simulink model "milestonetwo_oldsetup"  (R2025a)
settings: Solver=FixedStepAuto  StartTime=0.0  StopTime=10  FixedStep=1e-3  RelTol=1e-3  EnableMultiTasking=on
model workspace (MAT data in the model file):
  Var = 0
  x = 1
undefined symbols (not defined in the file): D0, D1, D10, D11, D12, D13, D2, D3, D5, D6, D8, D9, PTA0, PTA1, PTA2, PTB9, PTC16, PTC17, PTC2, PTC4, PTD0, PTD1, PTD2, PTD3
libraries: frdmk64flib x14
settings Model: ExtModeTrigDuration=5  Creator=alber  LastModifiedBy=ybakr
settings OptimizationCC: BlockReduction=off  DefaultParameterBehavior=Inlined  BufferReuse=off  EnhancedBackFolding=on  PassReuseOutputArgsAs=Individual arguments  ZeroExternalMemoryAtStartup=off  ZeroInternalMemoryAtStartup=off  MaxStackSize=64  OptimizeBlockOrder=speed  DifferentSizesBufferReuse=on  EfficientTunableParamExpr=on
settings DebuggingCC: ParameterTunabilityLossMsg=error
settings HardwareCC: ProdBitPerPointer=32.0  ProdBitPerSizeT=32.0  ProdBitPerPtrDiffT=32.0  ProdLargestAtomicInteger=Long  ProdLargestAtomicFloat=Double  ProdWordSize=32.0  ProdHWDeviceType=ARM Compatible->ARM Cortex
settings SFSimCC: MATLABDynamicMemAlloc=off
settings RTWCC: SystemTargetFile=ert.tlc  HardwareBoard=NXP FRDM-K64F  TLCOptions="-aInlineSetEventsForThisBaseRateFcn=TLC_FALSE -aSuppressMultiTaskScheduler=TLC_FALSE  -aRateBasedStepFcn=0"  TemplateMakefile=ert_default_tmf  Toolchain=GNU Tools for ARM Embedded Processors  Description=Embedded Coder
settings CodeAppCC: ForceParamTrailComments=on  IgnoreCustomStorageClasses=off  OperatorAnnotations=on  SimulinkDataObjDesc=on  SFDataObjDesc=on  InsertBlockDesc=on
settings ERTTargetCC: ExtModeTransport=4.0  ExtModeStaticAlloc=off  ExtModeMexFile=sendToCommService  ExtModeIntrfLevel=Level1

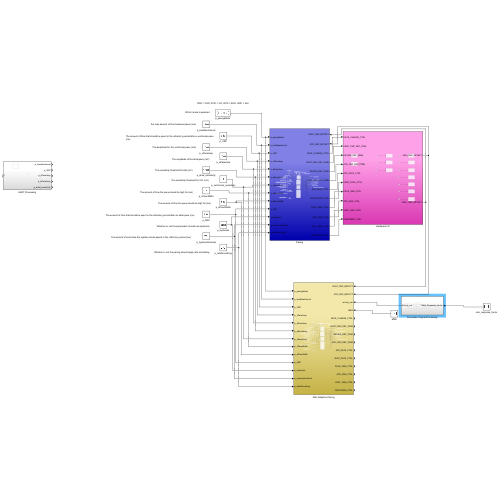
[thumbnail: Simulink's stored preview of the top-level diagram]
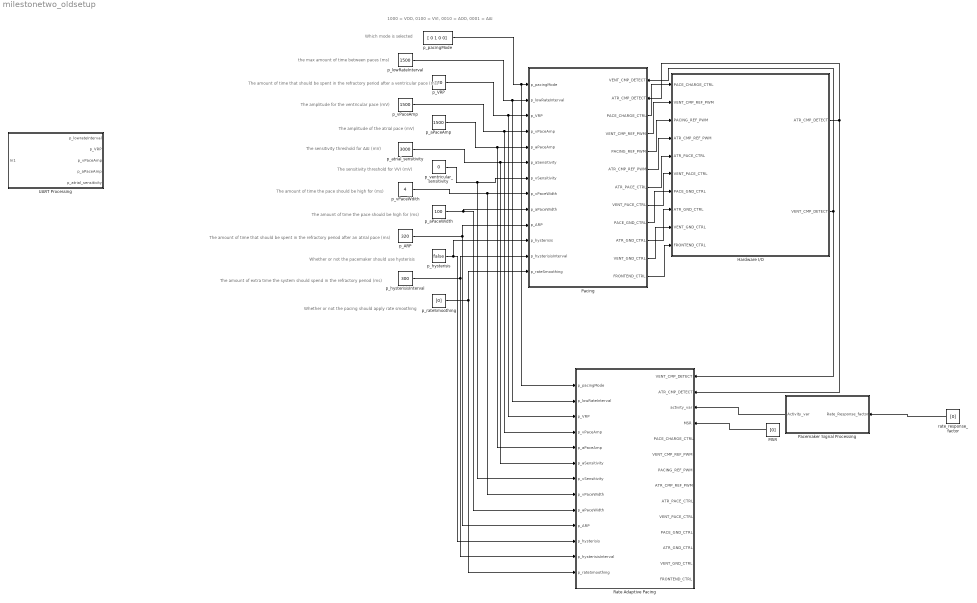
== system milestonetwo_oldsetup ==
  note: The amount of extra time the system should spend in the refractory period (ms)
  note: Whether or not the pacemaker should use hysterisis
  note: Whether or not the pacing should apply rate smoothing
  note: The amplitude of the atrial pace (mV)
  note: The sensitivity threshold for VVI (mV)
  note: The amount of time that should be spent in the refractory period after a ventricular pace (ms)
  note: The amount of time the pace should be high for (ms)
  note: The amplitude for the ventricular pace (mV)
  note: the max amount of time between paces (ms)
  note: Which mode is selected
  note: 1000 = VOO, 0100 = VVI, 0010 = AOO, 0001 = AAI
  note: The amount of time the pace should be high for (ms)
  note: The sensitivity threshold for AAI (mV)
  note: The amount of time that should be spent in the refractory period after an atrial pace (ms)
  Hardware I/O : Subsystem
  MSR : Constant  Value=[0]  OutDataTypeStr=uint16
  Pacemaker Signal Processing : Subsystem
  Pacing : Subsystem
      settings: PortSchema="{\"entries\":[{\"content\":{\"sides\":[{\"content\":{\"connectorIds\":[\"In1\",\"In2\",\"In3\",\"In4\",\"In5\",\"In6\",\"In7\",\"In8\",\"In9\",\"In10\",\"In11\",\"In12\",\"In13\"]},\"type\":\"ConnectorPlacement.EquallySpacedRectSide\",\"uuid\":\"83755f54-be08-4212-abd8-522318738612\"},{\"content\":{\"connectorIds\":[\"In14\",\"In15\",\"Out1\",\"Out2\",\"Out3\",\"Out4\",\"Out5\",\"Out6\",\"Out7\",\"Out8\",\"Out9\",\"Out10\"],\"side\":\"RIGHT\"},\"type\":\"ConnectorPlacement.EquallySpacedRectSide\",\"uuid\":\"fddfc3a4-50da-418e-a4c1-261999e6a94a\"},{\"content\":{\"side\":\"TOP\"},\"type\":\"ConnectorPlacement.EquallySpacedRectSide\",\"uuid\":\"96bf6691-7ea4-44be-8ce9-22c29429ec55\"}]},\"type\":\"ConnectorPlacement.EquallySpacedConnector\",\"uuid\":\"94865ebc-bf15-4e1f-8273-6a484a8d613b\"}],\"packageUris\":[\"http://schema.mathworks.com/mf0/Connector/R2020b\"],\"version\":\"1.0\"}"
  Rate Adaptive Pacing : Subsystem
      settings: PortSchema="{\"entries\":[{\"content\":{\"sides\":[{\"content\":{\"connectorIds\":[\"In1\",\"In2\",\"In3\",\"In4\",\"In5\",\"In6\",\"In7\",\"In8\",\"In9\",\"In10\",\"In11\",\"In12\",\"In13\"]},\"type\":\"ConnectorPlacement.EquallySpacedRectSide\",\"uuid\":\"83755f54-be08-4212-abd8-522318738612\"},{\"content\":{\"connectorIds\":[\"In14\",\"In15\",\"In16\",\"In17\",\"Out1\",\"Out2\",\"Out3\",\"Out4\",\"Out5\",\"Out6\",\"Out7\",\"Out8\",\"Out9\",\"Out10\"],\"side\":\"RIGHT\"},\"type\":\"ConnectorPlacement.EquallySpacedRectSide\",\"uuid\":\"fddfc3a4-50da-418e-a4c1-261999e6a94a\"},{\"content\":{\"side\":\"TOP\"},\"type\":\"ConnectorPlacement.EquallySpacedRectSide\",\"uuid\":\"96bf6691-7ea4-44be-8ce9-22c29429ec55\"}]},\"type\":\"ConnectorPlacement.EquallySpacedConnector\",\"uuid\":\"94865ebc-bf15-4e1f-8273-6a484a8d613b\"}],\"packageUris\":[\"http://schema.mathworks.com/mf0/Connector/R2020b\"],\"version\":\"1.0\"}"
  UART Processing : Subsystem
  p_ARP : Constant  Value=320  OutMin=[150]  OutMax=[500]  OutDataTypeStr=uint16
  p_VRP : Constant  Value=320  OutMin=[150]  OutMax=[500]  OutDataTypeStr=uint16
  p_aPaceAmp : Constant  Value=1500  OutDataTypeStr=uint16
  p_aPaceWidth : Constant  Value=100  OutDataTypeStr=int16
  p_atrial_sensitivity : Constant  Value=3000  OutDataTypeStr=uint16
  p_hysterisis : Constant  Value=false  OutDataTypeStr=uint16
  p_hysterisisInterval : Constant  Value=300  OutDataTypeStr=uint16
  p_lowRateInterval : Constant  Value=1500  OutMin=[343]  OutMax=[2000]  OutDataTypeStr=uint16
  p_pacingMode : Constant  Value=[ 0 1 0 0]  OutDataTypeStr=uint8
  p_rateSmoothing : Constant  Value=[0]  OutDataTypeStr=uint16
  p_vPaceAmp : Constant  Value=1500  OutMin=[500]  OutMax=[7000]  OutDataTypeStr=uint16
  p_vPaceWdith : Constant  Value=4  OutMin=[1]  OutMax=[19]  OutDataTypeStr=int16
  p_ventricular_sensitivity : Constant  Value=0  OutDataTypeStr=uint16
  rate_response_factor : Constant  Value=[0]  OutDataTypeStr=uint16
  wires:
  p_pacingMode/1 -> Rate Adaptive Pacing/1(p_pacingMode), Pacing/1(p_pacingMode)
  p_aPaceWidth/1 -> Rate Adaptive Pacing/9(p_aPaceWidth), Pacing/9(p_aPaceWidth)
  p_aPaceAmp/1 -> Rate Adaptive Pacing/5(p_aPaceAmp), Pacing/5(p_aPaceAmp)
  p_lowRateInterval/1 -> Rate Adaptive Pacing/2(p_lowRateInterval), Pacing/2(p_lowRateInterval)
  p_vPaceAmp/1 -> Rate Adaptive Pacing/4(p_vPaceAmp), Pacing/4(p_vPaceAmp)
  p_vPaceWdith/1 -> Rate Adaptive Pacing/8(p_vPaceWidth), Pacing/8(p_vPaceWidth)
  p_hysterisis/1 -> Rate Adaptive Pacing/11(p_hysterisis), Pacing/11(p_hysterisis)
  p_hysterisisInterval/1 -> Rate Adaptive Pacing/12(p_hysterisisInterval), Pacing/12(p_hysterisisInterval)
  p_rateSmoothing/1 -> Pacing/13(p_rateSmoothing), Rate Adaptive Pacing/13(p_rateSmoothing)
  Pacing/1(PACE_CHARGE_CTRL) -> Hardware I/O/1(PACE_CHARGE_CTRL)
  p_VRP/1 -> Rate Adaptive Pacing/3(p_VRP), Pacing/3(p_VRP)
  p_ARP/1 -> Rate Adaptive Pacing/10(p_ARP), Pacing/10(p_ARP)
  Pacing/2(VENT_CMP_REF_PWM) -> Hardware I/O/2(VENT_CMP_REF_PWM)
  Pacing/3(PACING_REF_PWM) -> Hardware I/O/3(PACING_REF_PWM)
  Pacing/4(ATR_CMP_REF_PWM) -> Hardware I/O/4(ATR_CMP_REF_PWM)
  Pacing/10(FRONTEND_CTRL) -> Hardware I/O/10(FRONTEND_CTRL)
  Pacing/9(VENT_GND_CTRL) -> Hardware I/O/9(VENT_GND_CTRL)
  Pacing/8(ATR_GND_CTRL) -> Hardware I/O/8(ATR_GND_CTRL)
  Pacing/7(PACE_GND_CTRL) -> Hardware I/O/7(PACE_GND_CTRL)
  Pacing/6(VENT_PACE_CTRL) -> Hardware I/O/6(VENT_PACE_CTRL)
  Pacing/5(ATR_PACE_CTRL) -> Hardware I/O/5(ATR_PACE_CTRL)
  Hardware I/O/1(ATR_CMP_DETECT) -> Pacing/15(ATR_CMP_DETECT), Rate Adaptive Pacing/15(ATR_CMP_DETECT)
  Hardware I/O/2(VENT_CMP_DETECT) -> Pacing/14(VENT_CMP_DETECT), Rate Adaptive Pacing/14(VENT_CMP_DETECT)
  p_atrial_sensitivity/1 -> Rate Adaptive Pacing/6(p_aSensitivity), Pacing/6(p_aSensitivity)
  p_ventricular_sensitivity/1 -> Rate Adaptive Pacing/7(p_vSensitivity), Pacing/7(p_vSensitivity)
  rate_response_factor/1 -> Pacemaker Signal Processing/1(Rate_Response_factor)
  Pacemaker Signal Processing/1(Activity_var) -> Rate Adaptive Pacing/16(activity_var)
  MSR/1 -> Rate Adaptive Pacing/17(MSR)

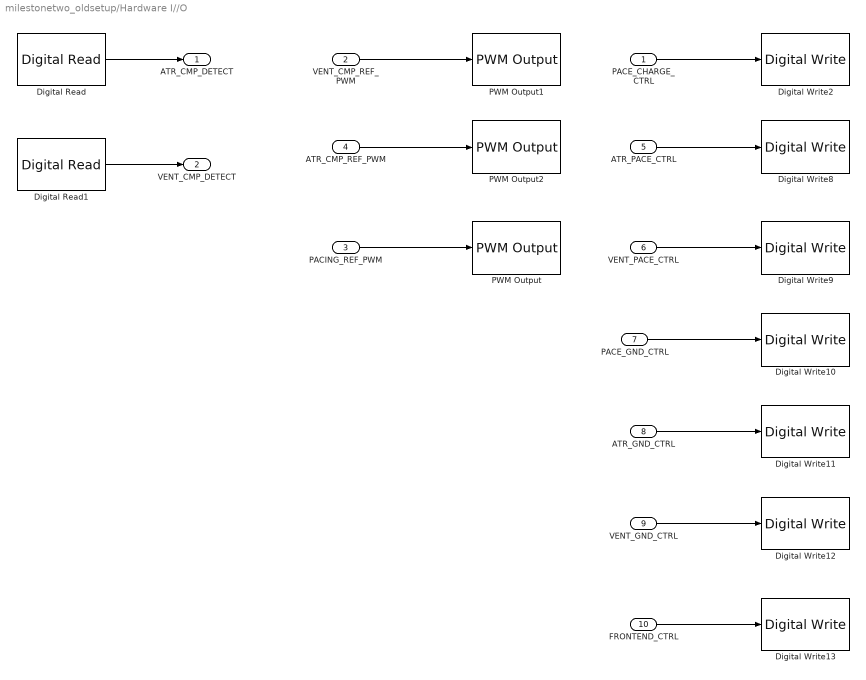
== system milestonetwo_oldsetup/Hardware I//O ==
  PACE_CHARGE_CTRL : Inport
  VENT_CMP_REF_PWM : Inport  Port=2
  PACING_REF_PWM : Inport  Port=3
  ATR_CMP_REF_PWM : Inport  Port=4
  ATR_PACE_CTRL : Inport  Port=5
  VENT_PACE_CTRL : Inport  Port=6
  PACE_GND_CTRL : Inport  Port=7
  ATR_GND_CTRL : Inport  Port=8
  VENT_GND_CTRL : Inport  Port=9
  FRONTEND_CTRL : Inport  Port=10
  Digital Read : frdmk64flib/Digital Read  Whichpin=PTC16 (D0)  SampleTime=-1
  Digital Read1 : frdmk64flib/Digital Read  Whichpin=PTC17 (D1)  SampleTime=-1
  Digital Write10 : frdmk64flib/Digital Write  Whichpin=PTD0 (D10)
  Digital Write11 : frdmk64flib/Digital Write  Whichpin=PTD2 (D11)
  Digital Write12 : frdmk64flib/Digital Write  Whichpin=PTD3 (D12)
  Digital Write13 : frdmk64flib/Digital Write  Whichpin=PTD1 (D13)
  Digital Write2 : frdmk64flib/Digital Write  Whichpin=PTB9 (D2)
  Digital Write8 : frdmk64flib/Digital Write  Whichpin=PTA0 (D8)
  Digital Write9 : frdmk64flib/Digital Write  Whichpin=PTC4 (D9)
  PWM Output : frdmk64flib/PWM Output  Whichpin=PTA2 (D5)  InitialFrequency=2000  InitialDutyCycle=0
  PWM Output1 : frdmk64flib/PWM Output  Whichpin=PTA1 (D3)  InitialFrequency=2000  InitialDutyCycle=0
  PWM Output2 : frdmk64flib/PWM Output  Whichpin=PTC2 (D6)  InitialFrequency=2000  InitialDutyCycle=0
  ATR_CMP_DETECT : Outport
  VENT_CMP_DETECT : Outport  Port=2
  wires:
  PACE_CHARGE_CTRL/1 -> Digital Write2/1
  PACING_REF_PWM/1 -> PWM Output/1
  VENT_CMP_REF_PWM/1 -> PWM Output1/1
  ATR_GND_CTRL/1 -> Digital Write11/1
  ATR_PACE_CTRL/1 -> Digital Write8/1
  VENT_PACE_CTRL/1 -> Digital Write9/1
  ATR_CMP_REF_PWM/1 -> PWM Output2/1
  VENT_GND_CTRL/1 -> Digital Write12/1
  FRONTEND_CTRL/1 -> Digital Write13/1
  Digital Read/1 -> ATR_CMP_DETECT/1
  Digital Read1/1 -> VENT_CMP_DETECT/1
  PACE_GND_CTRL/1 -> Digital Write10/1

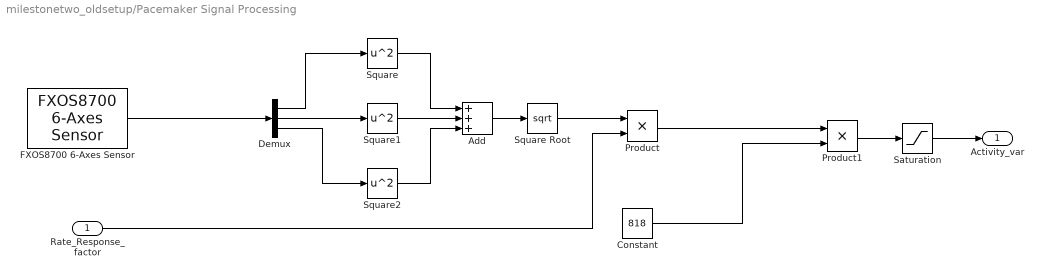
== system milestonetwo_oldsetup/Pacemaker Signal Processing ==
  Rate_Response_factor : Inport
  Add : Sum  Inputs=+++
  Constant : Constant  Value=818
  Demux : Demux  Outputs=3
  FXOS8700 6-Axes Sensor : frdmk64flib/FXOS8700 6-Axes Sensor  Activesensor=Accelerometer only  ODR=400Hz  HybridODR=400Hz  Accelfullrange=-4g to +4g  SampleTime=-1
  Product : Product
  Product1 : Product
  Saturation : Saturate  UpperLimit=7200  LowerLimit=1500
  Square : Math  Operator=square
  Square Root : Sqrt
  Square1 : Math  Operator=square
  Square2 : Math  Operator=square
  Activity_var : Outport
  wires:
  FXOS8700 6-Axes Sensor/1 -> Demux/1
  Rate_Response_factor/1 -> Product/2
  Demux/1 -> Square/1
  Demux/2 -> Square1/1
  Demux/3 -> Square2/1
  Square/1 -> Add/1
  Square1/1 -> Add/2
  Square2/1 -> Add/3
  Add/1 -> Square Root/1
  Square Root/1 -> Product/1
  Product/1 -> Product1/1
  Constant/1 -> Product1/2
  Product1/1 -> Saturation/1
  Saturation/1 -> Activity_var/1

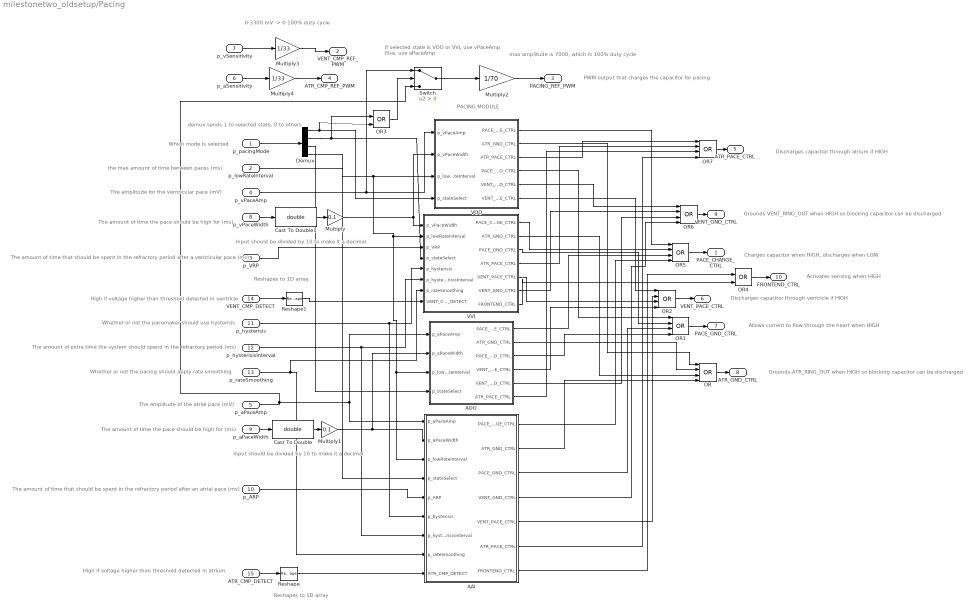
== system milestonetwo_oldsetup/Pacing ==
  note: Activates sensing when HIGH
  note: Charges capacitor when HIGH, discharges when LOW
  note: Allows current to flow through the heart when HIGH
  note: Grounds ATR_RING_OUT when HIGH so blocking capacitor can be discharged
  note: Discharges capacitor through ventricle if HIGH
  note: Grounds VENT_RING_OUT when HIGH so blocking capacitor can be discharged
  note: Discharges capacitor through atrium if HIGH
  note: PWM output that charges the capacitor for pacing
  note: High if voltage higher than threshold detected in atrium
  note: Input should be divided by 10 to make it a decimal
  note: Reshapes to 1D array
  note: demux sends 1 to selected state, 0 to others
  note: If selected state is VOO or VVI, use vPaceAmp
      | Else, use aPaceAmp
  note: max amplitude is 7000, which is 100% duty cycle
  note: 0-3300 mV -> 0-100% duty cycle
  note: PACING MODULE
  note: Reshapes to 1D array
  note: Input should be divided by 10 to make it a decimal
  note: Whether or not the pacing should apply rate smoothing
  note: the max amount of time between paces (ms)
  note: The amount of extra time the system should spend in the refractory period (ms)
  note: High if voltage higher than threshold detected in ventricle
  note: The amount of time the pace should be high for (ms)
  note: The amount of time the pace should be high for (ms)
  note: The amplitude of the atrial pace (mV)
  note: The amount of time that should be spent in the refractory period after a ventricular pace (ms)
  note: Whether or not the pacemaker should use hysterisis
  note: The amplitude for the ventricular pace (mV)
  note: The amount of time that should be spent in the refractory period after an atrial pace (ms)
  note: Which mode is selected
  p_pacingMode : Inport
  p_lowRateInterval : Inport  Port=2
  p_VRP : Inport  Port=3
  p_vPaceAmp : Inport  Port=4
  p_aPaceAmp : Inport  Port=5
  p_aSensitivity : Inport  Port=6
  p_vSensitivity : Inport  Port=7
  p_vPaceWidth : Inport  Port=8
  p_aPaceWidth : Inport  Port=9
  p_ARP : Inport  Port=10
  p_hysterisis : Inport  Port=11
  p_hysterisisInterval : Inport  Port=12
  p_rateSmoothing : Inport  Port=13
  VENT_CMP_DETECT : Inport  Port=14  OutDataTypeStr=boolean
  ATR_CMP_DETECT : Inport  Port=15  OutDataTypeStr=boolean
  AAI : Stateflow chart  TreatAsAtomicUnit=on
      settings: PortSchema="{\"entries\":[{\"content\":{\"sides\":[{\"content\":{\"connectorIds\":[\"In5\",\"In1\",\"In2\",\"In3\",\"In4\",\"In6\",\"In7\",\"In8\",\"In9\"]},\"type\":\"ConnectorPlacement.EquallySpacedRectSide\",\"uuid\":\"cccc9f32-b255-4089-8202-5f4b6cf4849a\"},{\"content\":{\"connectorIds\":[\"Out1\",\"Out2\",\"Out3\",\"Out4\",\"Out5\",\"Out6\",\"Out7\"],\"side\":\"RIGHT\"},\"type\":\"ConnectorPlacement.EquallySpacedRectSide\",\"uuid\":\"983a4a60-3d5c-4e53-84aa-b68c0bc6099e\"},{\"content\":{\"side\":\"TOP\"},\"type\":\"ConnectorPlacement.EquallySpacedRectSide\",\"uuid\":\"2756b790-cbb9-4039-b4f9-91cb14419ddd\"}]},\"type\":\"ConnectorPlacement.EquallySpacedConnector\",\"uuid\":\"1ccddf37-9dbc-46c0-8904-a3b9c6a38aa8\"}],\"packageUris\":[\"http://schema.mathworks.com/mf0/Connector/R2020b\"],\"version\":\"1.0\"}"
  AOO : Stateflow chart  TreatAsAtomicUnit=on
  Cast To Double : DataTypeConversion  OutDataTypeStr=double  SaturateOnIntegerOverflow=off  RndMeth=Floor
  Cast To Double1 : DataTypeConversion  OutDataTypeStr=double  SaturateOnIntegerOverflow=off  RndMeth=Floor
  Demux : Demux
  Multiply : Gain  Gain=0.1
  Multiply1 : Gain  Gain=0.1
  Multiply2 : Gain  Gain=1/70
  Multiply3 : Gain  Gain=1/33
  Multiply4 : Gain  Gain=1/33
  OR{,1..2,5..7} (6 alike) : Logic  Operator=OR  Inputs=4  IconShape=distinctive  AllPortsSameDT=off  OutDataTypeStr=boolean
  OR3 : Logic  Operator=OR  IconShape=distinctive  AllPortsSameDT=off  OutDataTypeStr=boolean
  OR4 : Logic  Operator=OR  IconShape=distinctive  AllPortsSameDT=off  OutDataTypeStr=boolean
  Reshape : Reshape
  Reshape1 : Reshape
  Switch : Switch  Criteria=u2 > Threshold  SaturateOnIntegerOverflow=off  InputSameDT=off
  VOO : Stateflow chart  TreatAsAtomicUnit=on
  VVI : Stateflow chart  TreatAsAtomicUnit=on
  PACE_CHARGE_CTRL : Outport
  VENT_CMP_REF_PWM : Outport  Port=2
  PACING_REF_PWM : Outport  Port=3
  ATR_CMP_REF_PWM : Outport  Port=4
  ATR_PACE_CTRL : Outport  Port=5
  VENT_PACE_CTRL : Outport  Port=6
  PACE_GND_CTRL : Outport  Port=7
  ATR_GND_CTRL : Outport  Port=8
  VENT_GND_CTRL : Outport  Port=9
  FRONTEND_CTRL : Outport  Port=10
  wires:
  Multiply/1 -> VVI/1(p_vPaceWidth), VOO/2(p_vPaceWidth)
  Multiply1/1 -> AAI/1(p_aPaceWidth), AOO/2(p_aPaceWidth)
  Cast To Double1/1 -> Multiply/1
  Cast To Double/1 -> Multiply1/1
  p_aPaceWidth/1 -> Cast To Double/1
  p_vPaceWidth/1 -> Cast To Double1/1
  p_lowRateInterval/1 -> AAI/2(p_lowRateInterval), AOO/3(p_lowRateInterval), VVI/2(p_lowRateInterval), VOO/3(p_lowRateInterval)
  p_ARP/1 -> AAI/4(p_ARP)
  p_VRP/1 -> VVI/3(p_VRP)
  p_hysterisis/1 -> AAI/6(p_hysterisis), VVI/5(p_hysterisis)
  p_hysterisisInterval/1 -> VVI/6(p_hysterisisInterval), AAI/7(p_hysterisisInterval)
  p_rateSmoothing/1 -> VVI/7(p_rateSmoothing), AAI/8(p_rateSmoothing)
  p_pacingMode/1 -> Demux/1
  Demux/1 -> OR3/2, VOO/4(p_stateSelect)
  Demux/2 -> OR3/1, VVI/4(p_stateSelect)
  Demux/3 -> AOO/4(p_stateSelect)
  Demux/4 -> AAI/3(p_stateSelect)
  p_vPaceAmp/1 -> Switch/1, VOO/1(p_vPaceAmp)
  p_aPaceAmp/1 -> AOO/1(p_aPaceAmp), AAI/5(p_aPaceAmp), Switch/3
  VOO/1(PACE_CHARGE_CTRL) -> OR5/1
  VVI/1(PACE_CHARGE_CTRL) -> OR5/2
  AOO/1(PACE_CHARGE_CTRL) -> OR5/3
  AAI/1(PACE_CHARGE_CTRL) -> OR5/4
  VOO/3(ATR_PACE_CTRL) -> OR7/1
  VVI/4(ATR_PACE_CTRL) -> OR7/2
  AOO/6(ATR_PACE_CTRL) -> OR7/3
  AOO/4(VENT_PACE_CTRL) -> OR2/4
  AAI/5(VENT_PACE_CTRL) -> OR2/2
  VVI/5(VENT_PACE_CTRL) -> OR2/3
  VOO/6(VENT_PACE_CTRL) -> OR2/1
  AAI/3(PACE_GND_CTRL) -> OR1/3
  AOO/3(PACE_GND_CTRL) -> OR1/4
  VVI/3(PACE_GND_CTRL) -> OR1/2
  VOO/4(PACE_GND_CTRL) -> OR1/1
  AAI/2(ATR_GND_CTRL) -> OR/4
  AOO/2(ATR_GND_CTRL) -> OR/2
  VVI/2(ATR_GND_CTRL) -> OR/3
  VOO/2(ATR_GND_CTRL) -> OR/1
  VOO/5(VENT_GND_CTRL) -> OR6/1
  VVI/6(VENT_GND_CTRL) -> OR6/2
  AOO/5(VENT_GND_CTRL) -> OR6/3
  AAI/4(VENT_GND_CTRL) -> OR6/4
  VVI/7(FRONTEND_CTRL) -> OR4/2
  AAI/7(FRONTEND_CTRL) -> OR4/1
  ATR_CMP_DETECT/1 -> Reshape/1
  VENT_CMP_DETECT/1 -> Reshape1/1
  Multiply2/1 -> PACING_REF_PWM/1
  Reshape/1 -> AAI/9(ATR_CMP_DETECT)
  Reshape1/1 -> VVI/8(VENT_CMP_DETECT)
  OR/1 -> ATR_GND_CTRL/1
  OR1/1 -> PACE_GND_CTRL/1
  OR2/1 -> VENT_PACE_CTRL/1
  OR3/1 -> Switch/2
  OR4/1 -> FRONTEND_CTRL/1
  OR5/1 -> PACE_CHARGE_CTRL/1
  OR6/1 -> VENT_GND_CTRL/1
  AAI/6(ATR_PACE_CTRL) -> OR7/4
  OR7/1 -> ATR_PACE_CTRL/1
  p_vSensitivity/1 -> Multiply3/1
  Multiply3/1 -> VENT_CMP_REF_PWM/1
  p_aSensitivity/1 -> Multiply4/1
  Multiply4/1 -> ATR_CMP_REF_PWM/1
  Switch/1 -> Multiply2/1

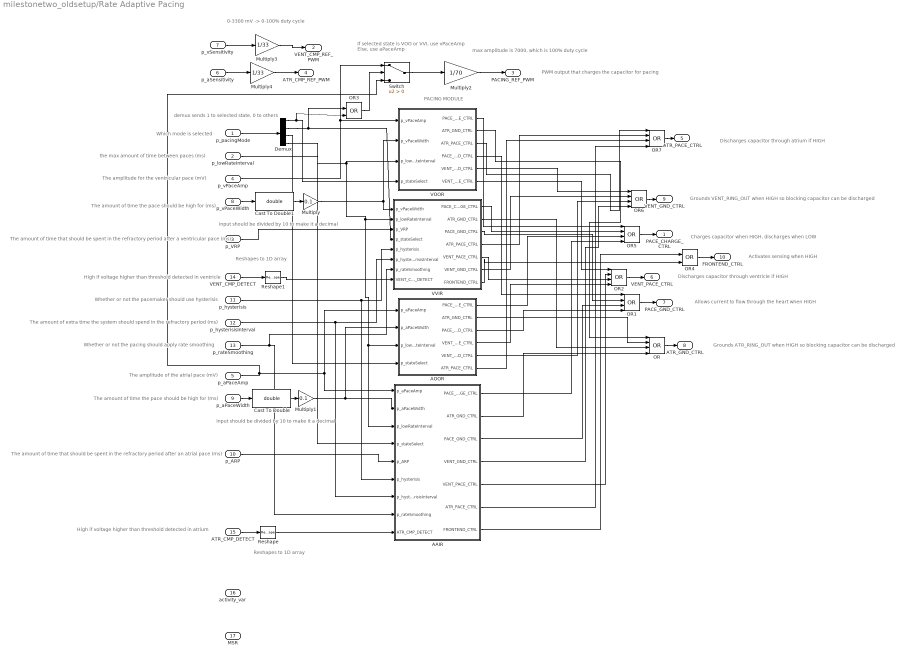
== system milestonetwo_oldsetup/Rate Adaptive Pacing ==
  note: Activates sensing when HIGH
  note: Charges capacitor when HIGH, discharges when LOW
  note: Allows current to flow through the heart when HIGH
  note: Grounds ATR_RING_OUT when HIGH so blocking capacitor can be discharged
  note: Discharges capacitor through ventricle if HIGH
  note: Grounds VENT_RING_OUT when HIGH so blocking capacitor can be discharged
  note: Discharges capacitor through atrium if HIGH
  note: PWM output that charges the capacitor for pacing
  note: High if voltage higher than threshold detected in atrium
  note: Input should be divided by 10 to make it a decimal
  note: Reshapes to 1D array
  note: demux sends 1 to selected state, 0 to others
  note: If selected state is VOO or VVI, use vPaceAmp
      | Else, use aPaceAmp
  note: max amplitude is 7000, which is 100% duty cycle
  note: 0-3300 mV -> 0-100% duty cycle
  note: PACING MODULE
  note: Reshapes to 1D array
  note: Input should be divided by 10 to make it a decimal
  note: Whether or not the pacing should apply rate smoothing
  note: the max amount of time between paces (ms)
  note: The amount of extra time the system should spend in the refractory period (ms)
  note: High if voltage higher than threshold detected in ventricle
  note: The amount of time the pace should be high for (ms)
  note: The amount of time the pace should be high for (ms)
  note: The amplitude of the atrial pace (mV)
  note: The amount of time that should be spent in the refractory period after a ventricular pace (ms)
  note: Whether or not the pacemaker should use hysterisis
  note: The amplitude for the ventricular pace (mV)
  note: The amount of time that should be spent in the refractory period after an atrial pace (ms)
  note: Which mode is selected
  p_pacingMode : Inport
  p_lowRateInterval : Inport  Port=2
  p_VRP : Inport  Port=3
  p_vPaceAmp : Inport  Port=4
  p_aPaceAmp : Inport  Port=5
  p_aSensitivity : Inport  Port=6
  p_vSensitivity : Inport  Port=7
  p_vPaceWidth : Inport  Port=8
  p_aPaceWidth : Inport  Port=9
  p_ARP : Inport  Port=10
  p_hysterisis : Inport  Port=11
  p_hysterisisInterval : Inport  Port=12
  p_rateSmoothing : Inport  Port=13
  VENT_CMP_DETECT : Inport  Port=14  OutDataTypeStr=boolean
  ATR_CMP_DETECT : Inport  Port=15  OutDataTypeStr=boolean
  activity_var : Inport  Port=16  OutDataTypeStr=boolean
  MSR : Inport  Port=17  OutDataTypeStr=boolean
  AAIR : Stateflow chart  TreatAsAtomicUnit=on
      settings: PortSchema="{\"entries\":[{\"content\":{\"sides\":[{\"content\":{\"connectorIds\":[\"In5\",\"In1\",\"In2\",\"In3\",\"In4\",\"In6\",\"In7\",\"In8\",\"In9\"]},\"type\":\"ConnectorPlacement.EquallySpacedRectSide\",\"uuid\":\"cccc9f32-b255-4089-8202-5f4b6cf4849a\"},{\"content\":{\"connectorIds\":[\"Out1\",\"Out2\",\"Out3\",\"Out4\",\"Out5\",\"Out6\",\"Out7\"],\"side\":\"RIGHT\"},\"type\":\"ConnectorPlacement.EquallySpacedRectSide\",\"uuid\":\"983a4a60-3d5c-4e53-84aa-b68c0bc6099e\"},{\"content\":{\"side\":\"TOP\"},\"type\":\"ConnectorPlacement.EquallySpacedRectSide\",\"uuid\":\"2756b790-cbb9-4039-b4f9-91cb14419ddd\"}]},\"type\":\"ConnectorPlacement.EquallySpacedConnector\",\"uuid\":\"1ccddf37-9dbc-46c0-8904-a3b9c6a38aa8\"}],\"packageUris\":[\"http://schema.mathworks.com/mf0/Connector/R2020b\"],\"version\":\"1.0\"}"
  AOOR : Stateflow chart  TreatAsAtomicUnit=on
  Cast To Double : DataTypeConversion  OutDataTypeStr=double  SaturateOnIntegerOverflow=off  RndMeth=Floor
  Cast To Double1 : DataTypeConversion  OutDataTypeStr=double  SaturateOnIntegerOverflow=off  RndMeth=Floor
  Demux : Demux
  Multiply : Gain  Gain=0.1
  Multiply1 : Gain  Gain=0.1
  Multiply2 : Gain  Gain=1/70
  Multiply3 : Gain  Gain=1/33
  Multiply4 : Gain  Gain=1/33
  OR{,1..2,5..7} (6 alike) : Logic  Operator=OR  Inputs=4  IconShape=distinctive  AllPortsSameDT=off  OutDataTypeStr=boolean
  OR3 : Logic  Operator=OR  IconShape=distinctive  AllPortsSameDT=off  OutDataTypeStr=boolean
  OR4 : Logic  Operator=OR  IconShape=distinctive  AllPortsSameDT=off  OutDataTypeStr=boolean
  Reshape : Reshape
  Reshape1 : Reshape
  Switch : Switch  Criteria=u2 > Threshold  SaturateOnIntegerOverflow=off  InputSameDT=off
  VOOR : Stateflow chart  TreatAsAtomicUnit=on
  VVIR : Stateflow chart  TreatAsAtomicUnit=on
  PACE_CHARGE_CTRL : Outport
  VENT_CMP_REF_PWM : Outport  Port=2
  PACING_REF_PWM : Outport  Port=3
  ATR_CMP_REF_PWM : Outport  Port=4
  ATR_PACE_CTRL : Outport  Port=5
  VENT_PACE_CTRL : Outport  Port=6
  PACE_GND_CTRL : Outport  Port=7
  ATR_GND_CTRL : Outport  Port=8
  VENT_GND_CTRL : Outport  Port=9
  FRONTEND_CTRL : Outport  Port=10
  wires:
  Multiply/1 -> VVIR/1(p_vPaceWidth), VOOR/2(p_vPaceWidth)
  Multiply1/1 -> AAIR/1(p_aPaceWidth), AOOR/2(p_aPaceWidth)
  Cast To Double1/1 -> Multiply/1
  Cast To Double/1 -> Multiply1/1
  p_aPaceWidth/1 -> Cast To Double/1
  p_vPaceWidth/1 -> Cast To Double1/1
  p_lowRateInterval/1 -> AAIR/2(p_lowRateInterval), AOOR/3(p_lowRateInterval), VVIR/2(p_lowRateInterval), VOOR/3(p_lowRateInterval)
  p_ARP/1 -> AAIR/4(p_ARP)
  p_VRP/1 -> VVIR/3(p_VRP)
  p_hysterisis/1 -> AAIR/6(p_hysterisis), VVIR/5(p_hysterisis)
  p_hysterisisInterval/1 -> VVIR/6(p_hysterisisInterval), AAIR/7(p_hysterisisInterval)
  p_rateSmoothing/1 -> VVIR/7(p_rateSmoothing), AAIR/8(p_rateSmoothing)
  p_pacingMode/1 -> Demux/1
  Demux/1 -> OR3/2, VOOR/4(p_stateSelect)
  Demux/2 -> OR3/1, VVIR/4(p_stateSelect)
  Demux/3 -> AOOR/4(p_stateSelect)
  Demux/4 -> AAIR/3(p_stateSelect)
  p_vPaceAmp/1 -> Switch/1, VOOR/1(p_vPaceAmp)
  p_aPaceAmp/1 -> AOOR/1(p_aPaceAmp), AAIR/5(p_aPaceAmp), Switch/3
  VOOR/1(PACE_CHARGE_CTRL) -> OR5/1
  VVIR/1(PACE_CHARGE_CTRL) -> OR5/2
  AOOR/1(PACE_CHARGE_CTRL) -> OR5/3
  AAIR/1(PACE_CHARGE_CTRL) -> OR5/4
  VOOR/3(ATR_PACE_CTRL) -> OR7/1
  VVIR/4(ATR_PACE_CTRL) -> OR7/2
  AOOR/6(ATR_PACE_CTRL) -> OR7/3
  AOOR/4(VENT_PACE_CTRL) -> OR2/4
  AAIR/5(VENT_PACE_CTRL) -> OR2/2
  VVIR/5(VENT_PACE_CTRL) -> OR2/3
  VOOR/6(VENT_PACE_CTRL) -> OR2/1
  AAIR/3(PACE_GND_CTRL) -> OR1/3
  AOOR/3(PACE_GND_CTRL) -> OR1/4
  VVIR/3(PACE_GND_CTRL) -> OR1/2
  VOOR/4(PACE_GND_CTRL) -> OR1/1
  AAIR/2(ATR_GND_CTRL) -> OR/4
  AOOR/2(ATR_GND_CTRL) -> OR/2
  VVIR/2(ATR_GND_CTRL) -> OR/3
  VOOR/2(ATR_GND_CTRL) -> OR/1
  VOOR/5(VENT_GND_CTRL) -> OR6/1
  VVIR/6(VENT_GND_CTRL) -> OR6/2
  AOOR/5(VENT_GND_CTRL) -> OR6/3
  AAIR/4(VENT_GND_CTRL) -> OR6/4
  VVIR/7(FRONTEND_CTRL) -> OR4/2
  AAIR/7(FRONTEND_CTRL) -> OR4/1
  ATR_CMP_DETECT/1 -> Reshape/1
  VENT_CMP_DETECT/1 -> Reshape1/1
  Multiply2/1 -> PACING_REF_PWM/1
  Reshape/1 -> AAIR/9(ATR_CMP_DETECT)
  Reshape1/1 -> VVIR/8(VENT_CMP_DETECT)
  OR/1 -> ATR_GND_CTRL/1
  OR1/1 -> PACE_GND_CTRL/1
  OR2/1 -> VENT_PACE_CTRL/1
  OR3/1 -> Switch/2
  OR4/1 -> FRONTEND_CTRL/1
  OR5/1 -> PACE_CHARGE_CTRL/1
  OR6/1 -> VENT_GND_CTRL/1
  AAIR/6(ATR_PACE_CTRL) -> OR7/4
  OR7/1 -> ATR_PACE_CTRL/1
  p_vSensitivity/1 -> Multiply3/1
  Multiply3/1 -> VENT_CMP_REF_PWM/1
  p_aSensitivity/1 -> Multiply4/1
  Multiply4/1 -> ATR_CMP_REF_PWM/1
  Switch/1 -> Multiply2/1

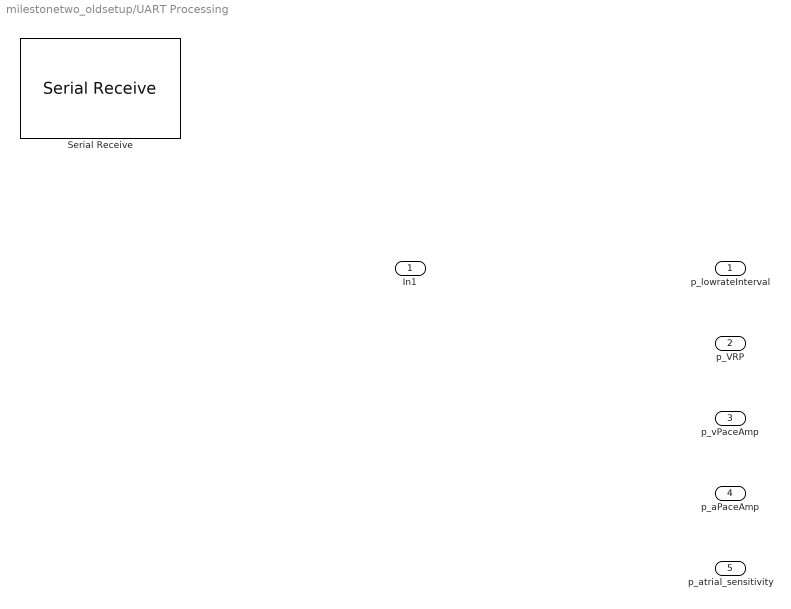
== system milestonetwo_oldsetup/UART Processing ==
  In1 : Inport
  Serial Receive : frdmk64flib/Serial Receive  SCIModule=0  Baudrate=uint32(9600)  Parity=None  StopBits=1  HardwareFlowControl=None  ByteOrder=LittleEndian  DataType=uint8  DataLength=10  BlockingMode=off  OutputStatus=on  SampleTime=0.1
  p_lowrateInterval : Outport
  p_VRP : Outport  Port=2
  p_vPaceAmp : Outport  Port=3
  p_aPaceAmp : Outport  Port=4
  p_atrial_sensitivity : Outport  Port=5

== stateflow chart milestonetwo_oldsetup/Pacing/VVI ==
  state REFRACTORY
    entry:
    current_state = "VVI REFRACTORY"
    FRONTEND_CTRL = 1;
    PACE_CHARGE_CTRL = 1;
    % Stop generating pace
    %Discharging blocking capacitor
    PACE_GND_CTRL = 1;
    VENT_PACE_CTRL = 0;
    ATR_PACE_CTRL = 0;
    ATR_GND_CTRL = 0;
    VENT_GND_CTRL = 1;
    %Charging C22
    %Would have to add a line here to update PWM when amplitude is able to be changed
    % Wait for a refractory period
    f_waitInterval = p_VRP; %p_hysterisis*p_hysterisisInterval
    if ~p_rateSmoothing == 0
    % Apply rate smoothing if enabled
    delta = f_waitInterval - prevInterval;
    maxDelta = (p_rateSmoothing / 100) * prevInterval; %Percent Rate Smoothing
    if abs(delta) > maxDelta
    delta = maxDelta;
    end
    nextInterval = prevInterval + delta;
    prevInterval = nextInterval;
    end
  state PACING
    entry:
    current_state = "VVI PACING"
    % Generate pace
    FRONTEND_CTRL = 0;
    PACE_CHARGE_CTRL = 0;
    VENT_PACE_CTRL = 1;
    PACE_GND_CTRL = 1;
    VENT_GND_CTRL = 0;
  note: VVI
  note: Stateflow cycles in INACTIVE when not selected
  state SENSING
    entry:
    current_state = "VVI SENSING"
    if ~isInitialized
    prevInterval = p_lowRateInterval;
    nextInterval = p_lowRateInterval;
    isInitialized = true;
    end
    test = VENT_CMP_DETECT
    FRONTEND_CTRL = 1;
    PACE_CHARGE_CTRL = 1;
    PACE_GND_CTRL = 1;
    VENT_PACE_CTRL = 0;
    ATR_PACE_CTRL = 0;
    ATR_GND_CTRL = 0;
    VENT_GND_CTRL = 1;
    % If the input signal is higher than the
    % sensitivity threshold, wait for another
    % refractory period
    % If the low rate interval passes and no
    % signals higher than the threshold are
    % detected, send another pace
  state INACTIVE
    % When stateflow isn't selected
  state hehe
    after(p_lowRateInterval-p_vPaceWidth-p_VRP, msec)
  PACING -> REFRACTORY : [after(p_vPaceWidth, msec)]
  (default) -> INACTIVE
  SENSING -> PACING [order 3] : [[after(p_lowRateInterval-p_vPaceWidth-p_VRP, msec)]]
  INACTIVE -> SENSING [order 1] : [p_stateSelect == 1]
  hehe -> REFRACTORY
  SENSING -> hehe [order 2] : [VENT_CMP_DETECT == 1]
  SENSING -> INACTIVE [order 1] : [p_stateSelect == 0]
  INACTIVE -> INACTIVE [order 2] : [p_stateSelect == 0]
  REFRACTORY -> SENSING : [after(f_waitInterval, msec)]
  data: p_vPaceWidth input double =0.4; p_lowRateInterval input uint16 =6000/low_rate_lim; p_VRP input uint16; p_stateSelect input uint8; current_state local string; p_hysterisis input; p_hysterisisInterval input; p_rateSmoothing input; delta local; f_waitInterval local; isInitialized local boolean =false; maxDelta local; nextInterval local; prevInterval local; PACE_CHARGE_CTRL output double; ATR_GND_CTRL output double; PACE_GND_CTRL output double; ATR_PACE_CTRL output double; VENT_PACE_CTRL output double; VENT_GND_CTRL output double; FRONTEND_CTRL output double; VENT_CMP_DETECT input boolean; test local

== stateflow chart milestonetwo_oldsetup/Pacing/AOO ==
  note: Max total cycle time - time already elapsed this cycle
  note: AOO Pacing Mode
  note: Cycle through this state when AoO isn't selected
  state CHARGE
    entry:
    % Output 0V
    current_state = "AOO CHARGE"
    %Discharging blocking capacitor
    PACE_GND_CTRL = 1;
    VENT_PACE_CTRL = 0;
    ATR_PACE_CTRL = 0;
    VENT_GND_CTRL = 0;
    ATR_GND_CTRL = 1; %DIFFERENT THAN DOC
    %Charging C22
    %Would have to add a line here to update PWM
    % When amplitude is able to be changed
    PACE_CHARGE_CTRL = 1;
  state PACE
    entry:
    % Output pace at specified amplitude
    current_state = "AOO PACE"
    PACE_CHARGE_CTRL = 0;
    PACE_GND_CTRL = 1;
    ATR_PACE_CTRL = 1;
    ATR_GND_CTRL = 0;
    VENT_GND_CTRL = 0;
    VENT_PACE_CTRL = 0;
    % Wait so that the pace has the specified width
  state INACTIVE
    % When state is not selected by input
  (default) -> INACTIVE
  CHARGE -> PACE [order 2] : [after(p_lowRateInterval - p_aPaceWidth, msec)]
  INACTIVE -> CHARGE [order 1] : [p_stateSelect == 1]
  CHARGE -> INACTIVE [order 1] : [p_stateSelect == 0]
  INACTIVE -> INACTIVE [order 2] : [p_stateSelect == 0]
  PACE -> CHARGE : after(p_aPaceWidth, msec)
  data: data local; p_aPaceAmp input uint16 =3500; p_aPaceWidth input double =0.4; p_lowRateInterval input uint16 =6000/low_rate_lim; p_stateSelect input uint8; current_state local string; PACE_CHARGE_CTRL output double; ATR_GND_CTRL output double; PACE_GND_CTRL output double; VENT_PACE_CTRL output double; VENT_GND_CTRL output double; ATR_PACE_CTRL output double

== stateflow chart milestonetwo_oldsetup/Pacing/VOO ==
  note: Total cycle time - time already elapsed this cycle
  note: VOO Pacing Mode
  state CHARGE
    entry:
    % Output 0V
    current_state = "VOO CHARGE"
    %Discharging blocking capacitor
    PACE_CHARGE_CTRL = 1;
    PACE_GND_CTRL = 1;
    VENT_PACE_CTRL = 0;
    ATR_PACE_CTRL = 0;
    ATR_GND_CTRL = 0;
    VENT_GND_CTRL = 1;
    %Charging C22
    %Would have to add a line here to update PWM
    % When amplitude is able to be changed
  state PACE
    entry:
    % Output pace at specified amplitude
    current_state = "VOO PACE"
    PACE_CHARGE_CTRL = 0;
    PACE_GND_CTRL = 1;
    ATR_PACE_CTRL = 0;
    ATR_GND_CTRL = 0;
    VENT_GND_CTRL = 0;
    VENT_PACE_CTRL = 1;
    % Wait so that the pace has the specified width
  state INACTIVE
    % Stateflow is inactive when not selected
  CHARGE -> PACE [order 2] : [after(p_lowRateInterval - p_vPaceWidth, msec)]
  (default) -> INACTIVE
  INACTIVE -> CHARGE [order 1] : [p_stateSelect == 1]
  CHARGE -> INACTIVE [order 1] : [p_stateSelect == 0]
  INACTIVE -> INACTIVE [order 2] : [p_stateSelect == 0]
  PACE -> CHARGE : after(p_vPaceWidth, msec)
  data: data local; p_vPaceAmp input uint16 =3500; p_vPaceWidth input double =0.4; p_lowRateInterval input uint16 =6000/low_rate_lim; p_stateSelect input uint8; current_state local string; PACE_CHARGE_CTRL output double; ATR_GND_CTRL output double; ATR_PACE_CTRL output double; PACE_GND_CTRL output double; VENT_GND_CTRL output double; VENT_PACE_CTRL output double

== stateflow chart milestonetwo_oldsetup/Pacing/AAI ==
  state PACING
    entry:
    state_out = "AAI PACING"
    FRONTEND_CTRL = 0;
    PACE_CHARGE_CTRL = 0;
    ATR_PACE_CTRL = 1;
    PACE_GND_CTRL = 1;
    ATR_GND_CTRL = 0;
    end
  state WAIT
    entry:
    state_out = "AAI SENSING"
    entry:
    if ~isInitialized
    prevInterval = p_lowRateInterval;
    nextInterval = p_lowRateInterval;
    isInitialized = true;
    end
    %Discharging blocking capacitor
    FRONTEND_CTRL = 1;
    PACE_CHARGE_CTRL = 1;
    PACE_GND_CTRL = 1;
    VENT_PACE_CTRL = 0;
    VENT_GND_CTRL = 0;
    ATR_PACE_CTRL = 0;
    ATR_GND_CTRL = 1; %DIFFERENT THAN DOC
    %Charging C22
    %Would have to add a line here to update PWM
    % When amplitude is able to be changed
  state INACTIVE
  state REFRACTORY
    entry:
    state_out = "AAI REFRACTORY"
    f_waitInterval = p_ARP% + p_hysterisis*p_hysterisisInterval;
    % Apply rate smoothing if enabled
    if ~p_rateSmoothing == 0
    delta = f_waitInterval - prevInterval;
    maxDelta = (p_rateSmoothing / 100) * prevInterval; %Percent Rate Smoothing
    if abs(delta) > maxDelta
    delta = maxDelta;
    end
    nextInterval = prevInterval + delta;
    prevInterval = nextInterval;
    end
    FRONTEND_CTRL = 1;
    PACE_CHARGE_CTRL = 1;
    PACE_GND_CTRL = 1;
    ATR_PACE_CTRL = 0;
    ATR_GND_CTRL = 1;
    VENT_GND_CTRL = 0;
    VENT_PACE_CTRL = 0;
    % Wait so that the pace has the specified width
  WAIT -> PACING [order 2] : [after(nextInterval,msec)]
  PACING -> REFRACTORY : [after(p_aPaceWidth, msec)]
  (default) -> INACTIVE
  INACTIVE -> WAIT [order 1] : [p_stateSelect == 1]
  WAIT -> INACTIVE [order 1] : [p_stateSelect == 0]
  INACTIVE -> INACTIVE [order 2] : [p_stateSelect == 0]
  WAIT -> REFRACTORY [order 3] : [ATR_CMP_DETECT == 1]
  REFRACTORY -> WAIT : [after(f_waitInterval,msec)]
  data: p_aPaceWidth input double =0.4; p_lowRateInterval input uint16 =6000/low_rate_lim; p_stateSelect input; p_ARP input; p_aPaceAmp input; p_hysterisis input; p_hysterisisInterval input; p_rateSmoothing input; delta local; f_waitInterval local; isInitialized local boolean =false; maxDelta local; nextInterval local; prevInterval local; state_out local string; PACE_CHARGE_CTRL output double; ATR_GND_CTRL output double; PACE_GND_CTRL output double; VENT_GND_CTRL output double; VENT_PACE_CTRL output double; ATR_PACE_CTRL output double; FRONTEND_CTRL output double; ATR_CMP_DETECT input boolean

== stateflow chart milestonetwo_oldsetup/Rate Adaptive Pacing/AAIR ==
  state PACING
    entry:
    state_out = "AAI PACING"
    FRONTEND_CTRL = 0;
    PACE_CHARGE_CTRL = 0;
    ATR_PACE_CTRL = 1;
    PACE_GND_CTRL = 1;
    ATR_GND_CTRL = 0;
    end
  state WAIT
    entry:
    state_out = "AAI SENSING"
    entry:
    if ~isInitialized
    prevInterval = p_lowRateInterval;
    nextInterval = p_lowRateInterval;
    isInitialized = true;
    end
    %Discharging blocking capacitor
    FRONTEND_CTRL = 1;
    PACE_CHARGE_CTRL = 1;
    PACE_GND_CTRL = 1;
    VENT_PACE_CTRL = 0;
    VENT_GND_CTRL = 0;
    ATR_PACE_CTRL = 0;
    ATR_GND_CTRL = 1; %DIFFERENT THAN DOC
    %Charging C22
    %Would have to add a line here to update PWM
    % When amplitude is able to be changed
  state INACTIVE
  state REFRACTORY
    entry:
    state_out = "AAI REFRACTORY"
    f_waitInterval = p_ARP + p_hysterisis*p_hysterisisInterval;
    % Apply rate smoothing if enabled
    if ~p_rateSmoothing == 0
    delta = f_waitInterval - prevInterval;
    maxDelta = (p_rateSmoothing / 100) * prevInterval; %Percent Rate Smoothing
    if abs(delta) > maxDelta
    delta = maxDelta;
    end
    nextInterval = prevInterval + delta;
    prevInterval = nextInterval;
    end
    FRONTEND_CTRL = 1;
    PACE_CHARGE_CTRL = 1;
    PACE_GND_CTRL = 1;
    ATR_PACE_CTRL = 0;
    ATR_GND_CTRL = 1;
    VENT_GND_CTRL = 0;
    VENT_PACE_CTRL = 0;
    % Wait so that the pace has the specified width
  WAIT -> PACING [order 2] : [after(nextInterval,msec)]
  PACING -> REFRACTORY : [after(p_aPaceWidth, msec)]
  (default) -> INACTIVE
  INACTIVE -> WAIT [order 1] : [p_stateSelect == 1]
  WAIT -> INACTIVE [order 1] : [p_stateSelect == 0]
  INACTIVE -> INACTIVE [order 2] : [p_stateSelect == 0]
  WAIT -> REFRACTORY [order 3] : [ATR_CMP_DETECT == 1]
  REFRACTORY -> WAIT : [after(f_waitInterval,msec)]
  data: p_aPaceWidth input double =0.4; p_lowRateInterval input uint16 =6000/low_rate_lim; p_stateSelect input; p_ARP input; p_aPaceAmp input; p_hysterisis input; p_hysterisisInterval input; p_rateSmoothing input; delta local; f_waitInterval local; isInitialized local boolean =false; maxDelta local; nextInterval local; prevInterval local; state_out local string; PACE_CHARGE_CTRL output double; ATR_GND_CTRL output double; PACE_GND_CTRL output double; VENT_GND_CTRL output double; VENT_PACE_CTRL output double; ATR_PACE_CTRL output double; FRONTEND_CTRL output double; ATR_CMP_DETECT input boolean

== stateflow chart milestonetwo_oldsetup/Rate Adaptive Pacing/AOOR ==
  note: Max total cycle time - time already elapsed this cycle
  note: AOO Pacing Mode
  note: Cycle through this state when AoO isn't selected
  state CHARGE
    entry:
    % Output 0V
    current_state = "AOO CHARGE"
    %Discharging blocking capacitor
    PACE_GND_CTRL = 1;
    VENT_PACE_CTRL = 0;
    ATR_PACE_CTRL = 0;
    VENT_GND_CTRL = 0;
    ATR_GND_CTRL = 1; %DIFFERENT THAN DOC
    %Charging C22
    %Would have to add a line here to update PWM
    % When amplitude is able to be changed
    PACE_CHARGE_CTRL = 1;
  state PACE
    entry:
    % Output pace at specified amplitude
    current_state = "AOO PACE"
    PACE_CHARGE_CTRL = 0;
    PACE_GND_CTRL = 1;
    ATR_PACE_CTRL = 1;
    ATR_GND_CTRL = 0;
    VENT_GND_CTRL = 0;
    VENT_PACE_CTRL = 0;
    % Wait so that the pace has the specified width
  state INACTIVE
    % When state is not selected by input
  (default) -> INACTIVE
  CHARGE -> PACE [order 2] : [after(p_lowRateInterval - p_aPaceWidth, msec)]
  INACTIVE -> CHARGE [order 1] : [p_stateSelect == 1]
  CHARGE -> INACTIVE [order 1] : [p_stateSelect == 0]
  INACTIVE -> INACTIVE [order 2] : [p_stateSelect == 0]
  PACE -> CHARGE : after(p_aPaceWidth, msec)
  data: data local; p_aPaceAmp input uint16 =3500; p_aPaceWidth input double =0.4; p_lowRateInterval input uint16 =6000/low_rate_lim; p_stateSelect input uint8; current_state local string; PACE_CHARGE_CTRL output double; ATR_GND_CTRL output double; PACE_GND_CTRL output double; VENT_PACE_CTRL output double; VENT_GND_CTRL output double; ATR_PACE_CTRL output double

== stateflow chart milestonetwo_oldsetup/Rate Adaptive Pacing/VOOR ==
  note: Total cycle time - time already elapsed this cycle
  note: VOO Pacing Mode
  state CHARGE
    entry:
    % Output 0V
    current_state = "VOO CHARGE"
    %Discharging blocking capacitor
    PACE_CHARGE_CTRL = 1;
    PACE_GND_CTRL = 1;
    VENT_PACE_CTRL = 0;
    ATR_PACE_CTRL = 0;
    ATR_GND_CTRL = 0;
    VENT_GND_CTRL = 1;
    %Charging C22
    %Would have to add a line here to update PWM
    % When amplitude is able to be changed
  state PACE
    entry:
    % Output pace at specified amplitude
    current_state = "VOO PACE"
    PACE_CHARGE_CTRL = 0;
    PACE_GND_CTRL = 1;
    ATR_PACE_CTRL = 0;
    ATR_GND_CTRL = 0;
    VENT_GND_CTRL = 0;
    VENT_PACE_CTRL = 1;
    % Wait so that the pace has the specified width
  state INACTIVE
    % Stateflow is inactive when not selected
  CHARGE -> PACE [order 2] : [after(p_lowRateInterval - p_vPaceWidth, msec)]
  (default) -> INACTIVE
  INACTIVE -> CHARGE [order 1] : [p_stateSelect == 1]
  CHARGE -> INACTIVE [order 1] : [p_stateSelect == 0]
  INACTIVE -> INACTIVE [order 2] : [p_stateSelect == 0]
  PACE -> CHARGE : after(p_vPaceWidth, msec)
  data: data local; p_vPaceAmp input uint16 =3500; p_vPaceWidth input double =0.4; p_lowRateInterval input uint16 =6000/low_rate_lim; p_stateSelect input uint8; current_state local string; PACE_CHARGE_CTRL output double; ATR_GND_CTRL output double; ATR_PACE_CTRL output double; PACE_GND_CTRL output double; VENT_GND_CTRL output double; VENT_PACE_CTRL output double

== stateflow chart milestonetwo_oldsetup/Rate Adaptive Pacing/VVIR ==
  state REFRACTORY
    entry:
    current_state = "VVI REFRACTORY"
    FRONTEND_CTRL = 1;
    PACE_CHARGE_CTRL = 1;
    % Stop generating pace
    %Discharging blocking capacitor
    PACE_GND_CTRL = 1;
    VENT_PACE_CTRL = 0;
    ATR_PACE_CTRL = 0;
    ATR_GND_CTRL = 0;
    VENT_GND_CTRL = 1;
    %Charging C22
    %Would have to add a line here to update PWM when amplitude is able to be changed
    % Wait for a refractory period
    f_waitInterval = p_VRP + p_hysterisis*p_hysterisisInterval
    if ~p_rateSmoothing == 0
    % Apply rate smoothing if enabled
    delta = f_waitInterval - prevInterval;
    maxDelta = (p_rateSmoothing / 100) * prevInterval; %Percent Rate Smoothing
    if abs(delta) > maxDelta
    delta = maxDelta;
    end
    nextInterval = prevInterval + delta;
    prevInterval = nextInterval;
    end
  state PACING
    entry:
    current_state = "VVI PACING"
    % Generate pace
    FRONTEND_CTRL = 0;
    PACE_CHARGE_CTRL = 0;
    VENT_PACE_CTRL = 1;
    PACE_GND_CTRL = 1;
    VENT_GND_CTRL = 0;
  note: VVI
  note: Stateflow cycles in INACTIVE when not selected
  state SENSING
    entry:
    current_state = "VVI SENSING"
    if ~isInitialized
    prevInterval = p_lowRateInterval;
    nextInterval = p_lowRateInterval;
    isInitialized = true;
    end
    test = VENT_CMP_DETECT
    FRONTEND_CTRL = 1;
    PACE_CHARGE_CTRL = 1;
    PACE_GND_CTRL = 1;
    VENT_PACE_CTRL = 0;
    ATR_PACE_CTRL = 0;
    ATR_GND_CTRL = 0;
    VENT_GND_CTRL = 1;
    % If the input signal is higher than the
    % sensitivity threshold, wait for another
    % refractory period
    % If the low rate interval passes and no
    % signals higher than the threshold are
    % detected, send another pace
  state INACTIVE
    % When stateflow isn't selected
  state hehe
    after(p_lowRateInterval-p_vPaceWidth-p_VRP, msec)
  PACING -> REFRACTORY : [after(p_vPaceWidth, msec)]
  (default) -> INACTIVE
  SENSING -> PACING [order 3] : [[after(p_lowRateInterval-p_vPaceWidth-p_VRP, msec)]]
  INACTIVE -> SENSING [order 1] : [p_stateSelect == 1]
  REFRACTORY -> SENSING : [after(f_waitInterval, msec)]
  hehe -> REFRACTORY
  SENSING -> hehe [order 2] : [VENT_CMP_DETECT == 1]
  SENSING -> INACTIVE [order 1] : [p_stateSelect == 0]
  INACTIVE -> INACTIVE [order 2] : [p_stateSelect == 0]
  data: p_vPaceWidth input double =0.4; p_lowRateInterval input uint16 =6000/low_rate_lim; p_VRP input uint16; p_stateSelect input uint8; current_state local string; p_hysterisis input; p_hysterisisInterval input; p_rateSmoothing input; delta local; f_waitInterval local; isInitialized local boolean =false; maxDelta local; nextInterval local; prevInterval local; PACE_CHARGE_CTRL output double; ATR_GND_CTRL output double; PACE_GND_CTRL output double; ATR_PACE_CTRL output double; VENT_PACE_CTRL output double; VENT_GND_CTRL output double; FRONTEND_CTRL output double; VENT_CMP_DETECT input boolean; test local
